simulink model "Basic_3DoF_Delta_2021a"  (R2021a)
settings: Solver=ode4  StartTime=0.0  StopTime=time(end)  FixedStep=0.001  RelTol=1e-6
model workspace: external: MATLAB File robot_6kg_v4_EXa5_DataFile.m (data not in the file)
values from neighbouring files (symbols this model uses):
  IAB = (Im + IA + IB)    [Basic_3DoF_Delta_Dynamic_Param.m]    (also in RL5_6kg_Dynamic_Param.m)
  IABe = (Im + IA + IBe)    [Basic_3DoF_Delta_Dynamic_Param.m]
  lB = l1*(rho1*m1 + me)    [Basic_3DoF_Delta_Dynamic_Param.m]    (also in RL5_6kg_Dynamic_Param.m)
  lBe = l1*(m1/2 + me)    [Basic_3DoF_Delta_Dynamic_Param.m]
  mD = m3 + 3*m2 + 3*me    [Basic_3DoF_Delta_Dynamic_Param.m]    (also in RL5_6kg_Dynamic_Param.m = m3 + 3*m2 + 3*me + mls_a4_spi + mls_a5_spi + mls_a5_worm)
  rho2 = Sro2    [Basic_3DoF_Delta_Dynamic_Param.m]    (also in RL5_6kg_Dynamic_Param.m)
undefined symbols (not defined in the file or in its folder): Inertias, X, Y, Z
libraries: sm_lib x119, nesl_utility x19, eeGeneralControl x3, simulink x3
(part 4 of 4)

== system Basic_3DoF_Delta_2021a/RL5_1450_6kg_Delta_robot_3DoF_Version/a16_pin2 _RIGID ==
  ReferenceFrame : sm_lib/Frames and Transforms/Reference Frame
  Solid(4) : sm_lib/Body Elements/File Solid  Description=Pin  ExtGeomFileName=a16_pin.stp  UnitType=FromFile  ExtGeomFileUnits=m  StepReaderType=HEX  ExportConvexHullGeometry=off  InertiaType=Custom  Mass=Inertias.Solid(4).mass  MassUnits=kg  CenterOfMass=Inertias.Solid(4).CoM  CenterOfMassUnits=m  MomentsOfInertia=Inertias.Solid(4).MoI  MomentsOfInertiaUnits=kg*m^2  ProductsOfInertia=Inertias.Solid(4).PoI  ProductsOfInertiaUnits=kg*m^2  BasedOnType=Density  Density=7850  DensityUnits=kg/m^3  DoExposeReferenceFrame=on  SerializedFrames=<Frames/>  GraphicType=FromGeometry  MarkerShape=Sphere  MarkerSize=10  GraphicVisPropType=SimpleVisualProperties  GraphicDiffuseColor=[0.8 0.8 0.8]  GraphicSpecularColor=[0.5 0.5 0.5 1.0]  GraphicAmbientColor=[0.15 0.15 0.15 1.0]  GraphicEmissiveColor=[0.0 0.0 0.0 1.0]  GraphicShininess=75  GraphicOpacity=1
      settings: AttributesFormatString=|
      | "%<Description>"
      | Mass: %<Mass> [%<MassUnits>]
      | CoM: %<CenterOfMass> [%<CenterOfMassUnits>]
      | MoI: %<MomentsOfInertia> [%<MomentsOfInertiaUnits>]
      | PoI: %<ProductsOfInertia> [%<ProductsOfInertiaUnits>]
  Transform : sm_lib/Frames and Transforms/Rigid Transform  TranslationMethod=StandardAxis  TranslationStandardOffset=67.5  TranslationLengthUnit=mm  TranslationStandardAxis=+X  TranslationCartesianOffset=0  TranslationROffset=0  TranslationROffsetUnits=m  TranslationZOffset=0  TranslationZOffsetUnits=m  TranslationThetaOffset=0  TranslationThetaOffsetUnits=deg  RotationMethod=StandardAxis  RotationAngleUnits=rad  RotationStandardAxis=+Z  RotationAngle=0  RotationArbitraryAxis=0  FollAlignAxisA=+X  BaseAlignAxisA=+Y  FollAlignAxisB=+Y  BaseAlignAxisB=+Z  RotationSequenceAxes=FollowerAxes  RotationSequence=XYX  RotationSequenceAngles=[0 0 0]  RotationSequenceAnglesUnits=deg  RotationMatrix=[1 0 0; 0 1 0; 0 0 1]
  Transform1 : sm_lib/Frames and Transforms/Rigid Transform  TranslationMethod=StandardAxis  TranslationStandardOffset=67.5  TranslationLengthUnit=mm  TranslationStandardAxis=-X  TranslationCartesianOffset=0  TranslationROffset=0  TranslationROffsetUnits=m  TranslationZOffset=0  TranslationZOffsetUnits=m  TranslationThetaOffset=0  TranslationThetaOffsetUnits=deg  RotationMethod=StandardAxis  RotationAngleUnits=deg  RotationStandardAxis=+Y  RotationAngle=180  RotationArbitraryAxis=0  FollAlignAxisA=+X  BaseAlignAxisA=+Y  FollAlignAxisB=+Y  BaseAlignAxisB=+Z  RotationSequenceAxes=FollowerAxes  RotationSequence=XYX  RotationSequenceAngles=[0 0 0]  RotationSequenceAnglesUnits=deg  RotationMatrix=[1 0 0; 0 1 0; 0 0 1]
  Transform2 : sm_lib/Frames and Transforms/Rigid Transform  TranslationMethod=None  TranslationStandardOffset=0  TranslationLengthUnit=mm  TranslationStandardAxis=+Z  TranslationCartesianOffset=0  TranslationROffset=0  TranslationROffsetUnits=m  TranslationZOffset=0  TranslationZOffsetUnits=m  TranslationThetaOffset=0  TranslationThetaOffsetUnits=deg  RotationMethod=StandardAxis  RotationAngleUnits=deg  RotationStandardAxis=+Y  RotationAngle=90  RotationArbitraryAxis=0  FollAlignAxisA=+X  BaseAlignAxisA=+Y  FollAlignAxisB=+Y  BaseAlignAxisB=+Z  RotationSequenceAxes=FollowerAxes  RotationSequence=XYX  RotationSequenceAngles=[0 0 0]  RotationSequenceAnglesUnits=deg  RotationMatrix=[1 0 0; 0 1 0; 0 0 1]
  Center : PMIOPort  Side=Right
  Link 1 : PMIOPort  Port=2  Side=Left
  Link 2 : PMIOPort  Port=3  Side=Left
  connections:
  Transform2/RConn1 -- Center/RConn1
  Transform1/RConn1 -- Link 2/RConn1
  Transform/RConn1 -- Link 1/RConn1
  Transform1/LConn1 -- Solid(4)/RConn1 -- Transform/LConn1 -- ReferenceFrame/RConn1 -- Transform2/LConn1

== system Basic_3DoF_Delta_2021a/RL5_1450_6kg_Delta_robot_3DoF_Version/a16_pin3 _RIGID ==
  ReferenceFrame : sm_lib/Frames and Transforms/Reference Frame
  Solid(4) : sm_lib/Body Elements/File Solid  Description=Pin  ExtGeomFileName=a16_pin.stp  UnitType=FromFile  ExtGeomFileUnits=m  StepReaderType=HEX  ExportConvexHullGeometry=off  InertiaType=Custom  Mass=Inertias.Solid(4).mass  MassUnits=kg  CenterOfMass=Inertias.Solid(4).CoM  CenterOfMassUnits=m  MomentsOfInertia=Inertias.Solid(4).MoI  MomentsOfInertiaUnits=kg*m^2  ProductsOfInertia=Inertias.Solid(4).PoI  ProductsOfInertiaUnits=kg*m^2  BasedOnType=Density  Density=7850  DensityUnits=kg/m^3  DoExposeReferenceFrame=on  SerializedFrames=<Frames/>  GraphicType=FromGeometry  MarkerShape=Sphere  MarkerSize=10  GraphicVisPropType=SimpleVisualProperties  GraphicDiffuseColor=[0.8 0.8 0.8]  GraphicSpecularColor=[0.5 0.5 0.5 1.0]  GraphicAmbientColor=[0.15 0.15 0.15 1.0]  GraphicEmissiveColor=[0.0 0.0 0.0 1.0]  GraphicShininess=75  GraphicOpacity=1
      settings: AttributesFormatString=|
      | "%<Description>"
      | Mass: %<Mass> [%<MassUnits>]
      | CoM: %<CenterOfMass> [%<CenterOfMassUnits>]
      | MoI: %<MomentsOfInertia> [%<MomentsOfInertiaUnits>]
      | PoI: %<ProductsOfInertia> [%<ProductsOfInertiaUnits>]
  Transform : sm_lib/Frames and Transforms/Rigid Transform  TranslationMethod=StandardAxis  TranslationStandardOffset=67.5  TranslationLengthUnit=mm  TranslationStandardAxis=+X  TranslationCartesianOffset=0  TranslationROffset=0  TranslationROffsetUnits=m  TranslationZOffset=0  TranslationZOffsetUnits=m  TranslationThetaOffset=0  TranslationThetaOffsetUnits=deg  RotationMethod=StandardAxis  RotationAngleUnits=rad  RotationStandardAxis=+Z  RotationAngle=0  RotationArbitraryAxis=0  FollAlignAxisA=+X  BaseAlignAxisA=+Y  FollAlignAxisB=+Y  BaseAlignAxisB=+Z  RotationSequenceAxes=FollowerAxes  RotationSequence=XYX  RotationSequenceAngles=[0 0 0]  RotationSequenceAnglesUnits=deg  RotationMatrix=[1 0 0; 0 1 0; 0 0 1]
  Transform1 : sm_lib/Frames and Transforms/Rigid Transform  TranslationMethod=StandardAxis  TranslationStandardOffset=67.5  TranslationLengthUnit=mm  TranslationStandardAxis=-X  TranslationCartesianOffset=0  TranslationROffset=0  TranslationROffsetUnits=m  TranslationZOffset=0  TranslationZOffsetUnits=m  TranslationThetaOffset=0  TranslationThetaOffsetUnits=deg  RotationMethod=StandardAxis  RotationAngleUnits=deg  RotationStandardAxis=+Y  RotationAngle=180  RotationArbitraryAxis=0  FollAlignAxisA=+X  BaseAlignAxisA=+Y  FollAlignAxisB=+Y  BaseAlignAxisB=+Z  RotationSequenceAxes=FollowerAxes  RotationSequence=XYX  RotationSequenceAngles=[0 0 0]  RotationSequenceAnglesUnits=deg  RotationMatrix=[1 0 0; 0 1 0; 0 0 1]
  Transform2 : sm_lib/Frames and Transforms/Rigid Transform  TranslationMethod=None  TranslationStandardOffset=0  TranslationLengthUnit=mm  TranslationStandardAxis=+Z  TranslationCartesianOffset=0  TranslationROffset=0  TranslationROffsetUnits=m  TranslationZOffset=0  TranslationZOffsetUnits=m  TranslationThetaOffset=0  TranslationThetaOffsetUnits=deg  RotationMethod=StandardAxis  RotationAngleUnits=deg  RotationStandardAxis=+Y  RotationAngle=90  RotationArbitraryAxis=0  FollAlignAxisA=+X  BaseAlignAxisA=+Y  FollAlignAxisB=+Y  BaseAlignAxisB=+Z  RotationSequenceAxes=FollowerAxes  RotationSequence=XYX  RotationSequenceAngles=[0 0 0]  RotationSequenceAnglesUnits=deg  RotationMatrix=[1 0 0; 0 1 0; 0 0 1]
  Center : PMIOPort  Side=Left
  Link 1 : PMIOPort  Port=2  Side=Right
  Link 2 : PMIOPort  Port=3  Side=Right
  connections:
  Transform2/RConn1 -- Center/RConn1
  Transform1/RConn1 -- Link 1/RConn1
  Transform/RConn1 -- Link 2/RConn1
  Transform/LConn1 -- Transform1/LConn1 -- Transform2/LConn1 -- Solid(4)/RConn1 -- ReferenceFrame/RConn1

== system Basic_3DoF_Delta_2021a/RL5_1450_6kg_Delta_robot_3DoF_Version/a16_pin4 _RIGID ==
  ReferenceFrame : sm_lib/Frames and Transforms/Reference Frame
  Solid(4) : sm_lib/Body Elements/File Solid  Description=Pin  ExtGeomFileName=a16_pin.stp  UnitType=FromFile  ExtGeomFileUnits=m  StepReaderType=HEX  ExportConvexHullGeometry=off  InertiaType=Custom  Mass=Inertias.Solid(4).mass  MassUnits=kg  CenterOfMass=Inertias.Solid(4).CoM  CenterOfMassUnits=m  MomentsOfInertia=Inertias.Solid(4).MoI  MomentsOfInertiaUnits=kg*m^2  ProductsOfInertia=Inertias.Solid(4).PoI  ProductsOfInertiaUnits=kg*m^2  BasedOnType=Density  Density=7850  DensityUnits=kg/m^3  DoExposeReferenceFrame=on  SerializedFrames=<Frames/>  GraphicType=FromGeometry  MarkerShape=Sphere  MarkerSize=10  GraphicVisPropType=SimpleVisualProperties  GraphicDiffuseColor=[0.8 0.8 0.8]  GraphicSpecularColor=[0.5 0.5 0.5 1.0]  GraphicAmbientColor=[0.15 0.15 0.15 1.0]  GraphicEmissiveColor=[0.0 0.0 0.0 1.0]  GraphicShininess=75  GraphicOpacity=1
      settings: AttributesFormatString=|
      | "%<Description>"
      | Mass: %<Mass> [%<MassUnits>]
      | CoM: %<CenterOfMass> [%<CenterOfMassUnits>]
      | MoI: %<MomentsOfInertia> [%<MomentsOfInertiaUnits>]
      | PoI: %<ProductsOfInertia> [%<ProductsOfInertiaUnits>]
  Transform : sm_lib/Frames and Transforms/Rigid Transform  TranslationMethod=StandardAxis  TranslationStandardOffset=67.5  TranslationLengthUnit=mm  TranslationStandardAxis=+X  TranslationCartesianOffset=0  TranslationROffset=0  TranslationROffsetUnits=m  TranslationZOffset=0  TranslationZOffsetUnits=m  TranslationThetaOffset=0  TranslationThetaOffsetUnits=deg  RotationMethod=StandardAxis  RotationAngleUnits=rad  RotationStandardAxis=+Z  RotationAngle=0  RotationArbitraryAxis=0  FollAlignAxisA=+X  BaseAlignAxisA=+Y  FollAlignAxisB=+Y  BaseAlignAxisB=+Z  RotationSequenceAxes=FollowerAxes  RotationSequence=XYX  RotationSequenceAngles=[0 0 0]  RotationSequenceAnglesUnits=deg  RotationMatrix=[1 0 0; 0 1 0; 0 0 1]
  Transform1 : sm_lib/Frames and Transforms/Rigid Transform  TranslationMethod=StandardAxis  TranslationStandardOffset=67.5  TranslationLengthUnit=mm  TranslationStandardAxis=-X  TranslationCartesianOffset=0  TranslationROffset=0  TranslationROffsetUnits=m  TranslationZOffset=0  TranslationZOffsetUnits=m  TranslationThetaOffset=0  TranslationThetaOffsetUnits=deg  RotationMethod=StandardAxis  RotationAngleUnits=deg  RotationStandardAxis=+Y  RotationAngle=180  RotationArbitraryAxis=0  FollAlignAxisA=+X  BaseAlignAxisA=+Y  FollAlignAxisB=+Y  BaseAlignAxisB=+Z  RotationSequenceAxes=FollowerAxes  RotationSequence=XYX  RotationSequenceAngles=[0 0 0]  RotationSequenceAnglesUnits=deg  RotationMatrix=[1 0 0; 0 1 0; 0 0 1]
  Transform2 : sm_lib/Frames and Transforms/Rigid Transform  TranslationMethod=None  TranslationStandardOffset=0  TranslationLengthUnit=mm  TranslationStandardAxis=+Z  TranslationCartesianOffset=0  TranslationROffset=0  TranslationROffsetUnits=m  TranslationZOffset=0  TranslationZOffsetUnits=m  TranslationThetaOffset=0  TranslationThetaOffsetUnits=deg  RotationMethod=StandardAxis  RotationAngleUnits=deg  RotationStandardAxis=+Y  RotationAngle=90  RotationArbitraryAxis=0  FollAlignAxisA=+X  BaseAlignAxisA=+Y  FollAlignAxisB=+Y  BaseAlignAxisB=+Z  RotationSequenceAxes=FollowerAxes  RotationSequence=XYX  RotationSequenceAngles=[0 0 0]  RotationSequenceAnglesUnits=deg  RotationMatrix=[1 0 0; 0 1 0; 0 0 1]
  Center : PMIOPort  Side=Right
  Link 1 : PMIOPort  Port=2  Side=Left
  Link 2 : PMIOPort  Port=3  Side=Left
  connections:
  Transform2/RConn1 -- Center/RConn1
  Transform1/RConn1 -- Link 2/RConn1
  Transform/RConn1 -- Link 1/RConn1
  Solid(4)/RConn1 -- Transform1/LConn1 -- Transform/LConn1 -- ReferenceFrame/RConn1 -- Transform2/LConn1

== system Basic_3DoF_Delta_2021a/RL5_1450_6kg_Delta_robot_3DoF_Version/a16_pin5 _RIGID ==
  ReferenceFrame : sm_lib/Frames and Transforms/Reference Frame
  Solid(4) : sm_lib/Body Elements/File Solid  Description=Pin  ExtGeomFileName=a16_pin.stp  UnitType=FromFile  ExtGeomFileUnits=m  StepReaderType=HEX  ExportConvexHullGeometry=off  InertiaType=Custom  Mass=Inertias.Solid(4).mass  MassUnits=kg  CenterOfMass=Inertias.Solid(4).CoM  CenterOfMassUnits=m  MomentsOfInertia=Inertias.Solid(4).MoI  MomentsOfInertiaUnits=kg*m^2  ProductsOfInertia=Inertias.Solid(4).PoI  ProductsOfInertiaUnits=kg*m^2  BasedOnType=Density  Density=7850  DensityUnits=kg/m^3  DoExposeReferenceFrame=on  SerializedFrames=<Frames/>  GraphicType=FromGeometry  MarkerShape=Sphere  MarkerSize=10  GraphicVisPropType=SimpleVisualProperties  GraphicDiffuseColor=[0.8 0.8 0.8]  GraphicSpecularColor=[0.5 0.5 0.5 1.0]  GraphicAmbientColor=[0.15 0.15 0.15 1.0]  GraphicEmissiveColor=[0.0 0.0 0.0 1.0]  GraphicShininess=75  GraphicOpacity=1
      settings: AttributesFormatString=|
      | "%<Description>"
      | Mass: %<Mass> [%<MassUnits>]
      | CoM: %<CenterOfMass> [%<CenterOfMassUnits>]
      | MoI: %<MomentsOfInertia> [%<MomentsOfInertiaUnits>]
      | PoI: %<ProductsOfInertia> [%<ProductsOfInertiaUnits>]
  Transform : sm_lib/Frames and Transforms/Rigid Transform  TranslationMethod=StandardAxis  TranslationStandardOffset=67.5  TranslationLengthUnit=mm  TranslationStandardAxis=+X  TranslationCartesianOffset=0  TranslationROffset=0  TranslationROffsetUnits=m  TranslationZOffset=0  TranslationZOffsetUnits=m  TranslationThetaOffset=0  TranslationThetaOffsetUnits=deg  RotationMethod=StandardAxis  RotationAngleUnits=rad  RotationStandardAxis=+Z  RotationAngle=0  RotationArbitraryAxis=0  FollAlignAxisA=+X  BaseAlignAxisA=+Y  FollAlignAxisB=+Y  BaseAlignAxisB=+Z  RotationSequenceAxes=FollowerAxes  RotationSequence=XYX  RotationSequenceAngles=[0 0 0]  RotationSequenceAnglesUnits=deg  RotationMatrix=[1 0 0; 0 1 0; 0 0 1]
  Transform1 : sm_lib/Frames and Transforms/Rigid Transform  TranslationMethod=StandardAxis  TranslationStandardOffset=67.5  TranslationLengthUnit=mm  TranslationStandardAxis=-X  TranslationCartesianOffset=0  TranslationROffset=0  TranslationROffsetUnits=m  TranslationZOffset=0  TranslationZOffsetUnits=m  TranslationThetaOffset=0  TranslationThetaOffsetUnits=deg  RotationMethod=StandardAxis  RotationAngleUnits=deg  RotationStandardAxis=+Y  RotationAngle=180  RotationArbitraryAxis=0  FollAlignAxisA=+X  BaseAlignAxisA=+Y  FollAlignAxisB=+Y  BaseAlignAxisB=+Z  RotationSequenceAxes=FollowerAxes  RotationSequence=XYX  RotationSequenceAngles=[0 0 0]  RotationSequenceAnglesUnits=deg  RotationMatrix=[1 0 0; 0 1 0; 0 0 1]
  Transform2 : sm_lib/Frames and Transforms/Rigid Transform  TranslationMethod=None  TranslationStandardOffset=0  TranslationLengthUnit=mm  TranslationStandardAxis=+Z  TranslationCartesianOffset=0  TranslationROffset=0  TranslationROffsetUnits=m  TranslationZOffset=0  TranslationZOffsetUnits=m  TranslationThetaOffset=0  TranslationThetaOffsetUnits=deg  RotationMethod=StandardAxis  RotationAngleUnits=deg  RotationStandardAxis=+Y  RotationAngle=90  RotationArbitraryAxis=0  FollAlignAxisA=+X  BaseAlignAxisA=+Y  FollAlignAxisB=+Y  BaseAlignAxisB=+Z  RotationSequenceAxes=FollowerAxes  RotationSequence=XYX  RotationSequenceAngles=[0 0 0]  RotationSequenceAnglesUnits=deg  RotationMatrix=[1 0 0; 0 1 0; 0 0 1]
  Center : PMIOPort  Side=Left
  Link 1 : PMIOPort  Port=2  Side=Right
  Link 2 : PMIOPort  Port=3  Side=Right
  connections:
  Transform2/RConn1 -- Center/RConn1
  Transform1/RConn1 -- Link 1/RConn1
  Transform/RConn1 -- Link 2/RConn1
  Transform/LConn1 -- Transform1/LConn1 -- Transform2/LConn1 -- Solid(4)/RConn1 -- ReferenceFrame/RConn1

== system Basic_3DoF_Delta_2021a/RL5_1450_6kg_Delta_robot_3DoF_Version/a16_pin6 _RIGID ==
  ReferenceFrame : sm_lib/Frames and Transforms/Reference Frame
  Solid(4) : sm_lib/Body Elements/File Solid  Description=Pin  ExtGeomFileName=a16_pin.stp  UnitType=FromFile  ExtGeomFileUnits=m  StepReaderType=HEX  ExportConvexHullGeometry=off  InertiaType=Custom  Mass=Inertias.Solid(4).mass  MassUnits=kg  CenterOfMass=Inertias.Solid(4).CoM  CenterOfMassUnits=m  MomentsOfInertia=Inertias.Solid(4).MoI  MomentsOfInertiaUnits=kg*m^2  ProductsOfInertia=Inertias.Solid(4).PoI  ProductsOfInertiaUnits=kg*m^2  BasedOnType=Density  Density=7850  DensityUnits=kg/m^3  DoExposeReferenceFrame=on  SerializedFrames=<Frames/>  GraphicType=FromGeometry  MarkerShape=Sphere  MarkerSize=10  GraphicVisPropType=SimpleVisualProperties  GraphicDiffuseColor=[0.8 0.8 0.8]  GraphicSpecularColor=[0.5 0.5 0.5 1.0]  GraphicAmbientColor=[0.15 0.15 0.15 1.0]  GraphicEmissiveColor=[0.0 0.0 0.0 1.0]  GraphicShininess=75  GraphicOpacity=1
      settings: AttributesFormatString=|
      | "%<Description>"
      | Mass: %<Mass> [%<MassUnits>]
      | CoM: %<CenterOfMass> [%<CenterOfMassUnits>]
      | MoI: %<MomentsOfInertia> [%<MomentsOfInertiaUnits>]
      | PoI: %<ProductsOfInertia> [%<ProductsOfInertiaUnits>]
  Transform : sm_lib/Frames and Transforms/Rigid Transform  TranslationMethod=StandardAxis  TranslationStandardOffset=67.5  TranslationLengthUnit=mm  TranslationStandardAxis=+X  TranslationCartesianOffset=0  TranslationROffset=0  TranslationROffsetUnits=m  TranslationZOffset=0  TranslationZOffsetUnits=m  TranslationThetaOffset=0  TranslationThetaOffsetUnits=deg  RotationMethod=StandardAxis  RotationAngleUnits=rad  RotationStandardAxis=+Z  RotationAngle=0  RotationArbitraryAxis=0  FollAlignAxisA=+X  BaseAlignAxisA=+Y  FollAlignAxisB=+Y  BaseAlignAxisB=+Z  RotationSequenceAxes=FollowerAxes  RotationSequence=XYX  RotationSequenceAngles=[0 0 0]  RotationSequenceAnglesUnits=deg  RotationMatrix=[1 0 0; 0 1 0; 0 0 1]
  Transform1 : sm_lib/Frames and Transforms/Rigid Transform  TranslationMethod=StandardAxis  TranslationStandardOffset=67.5  TranslationLengthUnit=mm  TranslationStandardAxis=-X  TranslationCartesianOffset=0  TranslationROffset=0  TranslationROffsetUnits=m  TranslationZOffset=0  TranslationZOffsetUnits=m  TranslationThetaOffset=0  TranslationThetaOffsetUnits=deg  RotationMethod=StandardAxis  RotationAngleUnits=deg  RotationStandardAxis=+Y  RotationAngle=180  RotationArbitraryAxis=0  FollAlignAxisA=+X  BaseAlignAxisA=+Y  FollAlignAxisB=+Y  BaseAlignAxisB=+Z  RotationSequenceAxes=FollowerAxes  RotationSequence=XYX  RotationSequenceAngles=[0 0 0]  RotationSequenceAnglesUnits=deg  RotationMatrix=[1 0 0; 0 1 0; 0 0 1]
  Transform2 : sm_lib/Frames and Transforms/Rigid Transform  TranslationMethod=None  TranslationStandardOffset=0  TranslationLengthUnit=mm  TranslationStandardAxis=+Z  TranslationCartesianOffset=0  TranslationROffset=0  TranslationROffsetUnits=m  TranslationZOffset=0  TranslationZOffsetUnits=m  TranslationThetaOffset=0  TranslationThetaOffsetUnits=deg  RotationMethod=StandardAxis  RotationAngleUnits=deg  RotationStandardAxis=+Y  RotationAngle=90  RotationArbitraryAxis=0  FollAlignAxisA=+X  BaseAlignAxisA=+Y  FollAlignAxisB=+Y  BaseAlignAxisB=+Z  RotationSequenceAxes=FollowerAxes  RotationSequence=XYX  RotationSequenceAngles=[0 0 0]  RotationSequenceAnglesUnits=deg  RotationMatrix=[1 0 0; 0 1 0; 0 0 1]
  Center : PMIOPort  Side=Right
  Link 1 : PMIOPort  Port=2  Side=Left
  Link 2 : PMIOPort  Port=3  Side=Left
  connections:
  Transform2/RConn1 -- Center/RConn1
  Transform1/RConn1 -- Link 2/RConn1
  Transform/RConn1 -- Link 1/RConn1
  Solid(4)/RConn1 -- Transform1/LConn1 -- Transform/LConn1 -- ReferenceFrame/RConn1 -- Transform2/LConn1

== matlab function Basic_3DoF_Delta_2021a/Dynamic Model ==
  data: Psi output; dD input; D input; q input; dq input; ddq input; dynpar input; tau_cp output; tau_ce output
function [Psi,tau_cp,tau_ce] = dyn(dD,D,q,dq,ddq,dynpar)
% This function block represents mathematical DYNAMIC MODEL for Basic 3-DoF Delta 

q0 = 5.327998*pi/180;   % [rad], 5.327998° ~ q0*pi/180 rad, angle( axis_i & line(A_i,B_i) )
r0 =  0.330;            % [m], radius of circumscribed circle of equilat. basic frame triangle
l1 =  0.420;            % [m], lengths of upper arms
% l2 =  1.055;          % [m], lengths of forearms, not used
r3 =  0.125;            % [m], radius of circumscribed circle of equilat. mov. platform trngl.
% r4 =  0.0632;         % [m], radius of wrist arm offset, distance from point E to F
% r4m = 0.0424798;      % [m], radius of wrist arm CoG point offset,distance from point E to \bar{F} 
% h4 =  0.132;          % [m], perpendicular distance from point D to E (h4m = h4), not used
% r5 =  0.135;          % [m], radius of swivel arm (distance A5-axis vs. Tool Center Point (TCP)), not used
% r5m = 0.1225 - 0.0432725;     % distance from F to the CoG of the swivel arm; translation in Z = 0.1225, Inertias.Solid(11).CoM(3)=0.0432725. 
dr =  r0 - r3;                  % [m], useful simplifying constant

% Actuated joint positions
q1 = q(1) - q0; q2 = q(2) - q0;  q3 = q(3) - q0;    % q4 = q(4);  q5 = q(5);

% Actuated joint velocities
dq1 = dq(1);  dq2 = dq(2);  dq3 = dq(3);            % dq4 = dq(4);  dq5 = dq(5);

% Actuated joint accelerations
ddq1 = ddq(1);  ddq2 = ddq(2);  ddq3 = ddq(3);      % ddq4 = ddq(4);  ddq5 = ddq(5);

% Point D positions
xD = D(1);  yD = D(2);  zD = D(3); 

% Point D velocities
dxD = dD(1);  dyD = dD(2);  dzD = dD(3);

%% Dynamic model mass parameters
g = 9.80665;        % [m]/s^2, gravity

mD = dynpar(1);     % Constant total mass at movable platform level (point D)

%% Jacobian matrices J_D, J_q, J_\mathcal{D} and their derivatives and inverses

[Jd,Jq] = Jcq(xD,yD,zD,dr,l1,q1,q2,q3);             % Eq (20) in the paper: Jd = J_D, Jq = J_q 
Jqd = Jd\Jq; iJqd = Jq\Jd;                          % Eq (21) in the paper: Jqd = J_qD, iJqd = J_qD^{-1}

JD = [Jqd, zeros(3,2); zeros(2,3), eye(2)];         % Eq (22) in the paper: JD = J_\mathcal{D}

[dJc,dJq] = dJcq(xD,yD,zD,dxD,dyD,dzD,dr,l1,q1,q2,q3,dq1,dq2,dq3); 
dJqd = Jd\(dJq-dJc*Jqd);                            % Eq (25) in the paper: derivative of J_qD

dJD = [dJqd, zeros(3,2) ; zeros(2,3), zeros(2)];    % derivative of J_\mathcal{D}

%% Dynamical model of the parallel part (A1-A2-A3): Equation of Motion: Eq. (40) with (51)

ld = sqrt(xD^2+yD^2);                   % distance of point D inn XY plane from point O

m2 = 1.05;
rho2 = dynpar(2);                       % mass distribution ratio for upper arms 
rho2e = 2/3;                            % in Codourey'96

mD =  mD - ( rho2*m2*(cos(q1)+cos(q2)+cos(q3)) );    % the mass of the movable platform with trajectoryy-dependent contribution of forearm masses
mDe = mD - 2*m2;                                     % in Codourey'96

IAB = dynpar(3);                                     % fixed inertia values of each upper arm excluding the effect of m2
IAB = diag([IAB + l1^2*rho2*cos(q1)*m2, IAB + l1^2*rho2*cos(q2)*m2, IAB + l1^2*rho2*cos(q3)*m2, 0, 0]); % inertia matrix for upper arms 
IABe = dynpar(5);                                    % in Codourey'96
IABe = diag([IABe + l1^2*rho2e*m2, IABe + l1^2*rho2e*m2, IABe + l1^2*rho2e*m2, 0, 0]); % in Codourey'96

I_35 = [eye(3), zeros(3,2)];
Ma = I_35*( IAB + mD*(JD'*JD) );        % Eq. (51) in the paper: Inertial matrix for the parallel part
Mae = I_35*( IABe + mDe*(JD'*JD) );     % in Codourey'96

Ca = I_35*( mD*JD'*dJD ) ;              % Eq. (51) in the paper: Coriolis & centrifugal matrix for the parallel part
Cae = I_35*( mDe*JD'*dJD ) ;            % in Codourey'96

lBnum = dynpar(4);
lBnume = dynpar(6); 

Ga = I_35*diag([lBnum + l1*rho2*cos(q1)*m2, lBnum + l1*rho2*cos(q2)*m2, lBnum + l1*rho2*cos(q3)*m2, 0, 0])*g*[cos(q1); cos(q2); cos(q3); 0; 0] ...
   - I_35*( mD*JD' )*[0; 0; -g; 0; 0] ;      % Eq. (51) with (48) in the paper: Gravitational matrix for the parallel part
Gae = I_35*diag([lBnume + l1*rho2e*m2, lBnume + l1*rho2e*m2, lBnume + l1*rho2e*m2, 0, 0])*g*[cos(q1); cos(q2); cos(q3); 0; 0] ...
   - I_35*( mDe*JD' )*[0; 0; -g; 0; 0] ;     % in Codourey'96


tau_ap = Ma*ddq + Ca*dq + Ga ;                                   % Torque vector of the actuated upper arms with proposed model
tau_ae = Mae*ddq + Cae*dq + Gae ;                                % with Coudrey'96 model

%% Collecting data for the regressor matrix (64) of the regression model from the sampled values of (62)
Sig10 = ddq1; 
% Sig14 = g*JF(3,1) + dq1*(dJF(1,1)*JF(1,1) + dJF(2,1)*JF(2,1) + dJF(3,1)*JF(3,1) + dJF(4,1)*JF(4,1)) + dq2*(dJF(1,2)*JF(1,1) + dJF(2,2)*JF(2,1) + dJF(3,2)*JF(3,1) + dJF(4,2)*JF(4,1)) + dq3*(dJF(1,3)*JF(1,1) + dJF(2,3)*JF(2,1) + dJF(3,3)*JF(3,1) + dJF(4,3)*JF(4,1)) + dq4*(dJF(1,4)*JF(1,1) + dJF(2,4)*JF(2,1) + dJF(3,4)*JF(3,1) + dJF(4,4)*JF(4,1)) + ddq1*(JF (1,1)^2 + JF (2,1)^2 + JF (3,1)^2 + JF (4,1)^2) + ddq2*(JF(1,1)*JF(1,2) + JF(2,1)*JF(2,2) + JF(3,1)*JF(3,2) + JF(4,1)*JF(4,2)) + ddq3*(JF(1,1)*JF(1,3) + JF(2,1)*JF(2,3) + JF(3,1)*JF(3,3) + JF(4,1)*JF(4,3)) + ddq4*(JF(1,1)*JF(1,4) + JF(2,1)*JF(2,4) + JF(3,1)*JF(3,4) + JF(4,1)*JF(4,4));
Sig14 = 0;      % due excluding wrist arm, i.e. m4=0
% Sig15 = g*JH(3,1) + dq1*(dJH(1,1)*JH(1,1) + dJH(2,1)*JH(2,1) + dJH(3,1)*JH(3,1) + dJH(4,1)*JH(4,1) + dJH(5,1)*JH(5,1)) + dq2*(dJH(1,2)*JH(1,1) + dJH(2,2)*JH(2,1) + dJH(3,2)*JH(3,1) + dJH(4,2)*JH(4,1) + dJH(5,2)*JH(5,1)) + dq3*(dJH(1,3)*JH(1,1) + dJH(2,3)*JH(2,1) + dJH(3,3)*JH(3,1) + dJH(4,3)*JH(4,1) + dJH(5,3)*JH(5,1)) + dq4*(dJH(1,4)*JH(1,1) + dJH(2,4)*JH(2,1) + dJH(3,4)*JH(3,1) + dJH(4,4)*JH(4,1) + dJH(5,4)*JH(5,1)) + dq5*(dJH(1,5)*JH(1,1) + dJH(2,5)*JH(2,1) + dJH(3,5)*JH(3,1) + dJH(4,5)*JH(4,1) + dJH(5,5)*JH(5,1)) + ddq1*(JH (1,1)^2 + JH (2,1)^2 + JH (3,1)^2 + JH (4,1)^2 + JH (5,1)^2) + ddq2*(JH(1,1)*JH(1,2) + JH(2,1)*JH(2,2) + JH(3,1)*JH(3,2) + JH(4,1)*JH(4,2) + JH(5,1)*JH(5,2)) + ddq3*(JH(1,1)*JH(1,3) + JH(2,1)*JH(2,3) + JH(3,1)*JH(3,3) + JH(4,1)*JH(4,3) + JH(5,1)*JH(5,3)) + ddq4*(JH(1,1)*JH(1,4) + JH(2,1)*JH(2,4) + JH(3,1)*JH(3,4) + JH(4,1)*JH(4,4) + JH(5,1)*JH(5,4)) + ddq5*(JH(1,1)*JH(1,5) + JH(2,1)*JH(2,5) + JH(3,1)*JH(3,5) + JH(4,1)*JH(4,5) + JH(5,1)*JH(5,5));
Sig15 = 0;      % due excluding swivel arm, i.e. m5=0
Sig1D = g*JD(3,1) + dq1*(dJqd(1,1)*JD(1,1) + dJqd(2,1)*JD(2,1) + dJqd(3,1)*JD(3,1)) + dq2*(dJqd(1,2)*JD(1,1) + dJqd(2,2)*JD(2,1) + dJqd(3,2)*JD(3,1)) + dq3*(dJqd(1,3)*JD(1,1) + dJqd(2,3)*JD(2,1) + dJqd(3,3)*JD(3,1)) + ddq1*(JD (1,1)^2 + JD (2,1)^2 + JD (3,1)^2) + ddq2*(JD(1,1)*JD(1,2) + JD(2,1)*JD(2,2) + JD(3,1)*JD(3,2)) + ddq3*(JD(1,1)*JD(1,3) + JD(2,1)*JD(2,3) + JD(3,1)*JD(3,3));
% Sig1Ds = g*JD(3,1);
Sig1Ds = 0;     % due excluding shafts, i.e. m6l=m6u=0 or mDs=0
%
Sig20 = ddq2; 
% Sig24 = g*JF(3,2) + dq1*(dJF(1,1)*JF(1,2) + dJF(2,1)*JF(2,2) + dJF(3,1)*JF(3,2) + dJF(4,1)*JF(4,2)) + dq2*(dJF(1,2)*JF(1,2) + dJF(2,2)*JF(2,2) + dJF(3,2)*JF(3,2) + dJF(4,2)*JF(4,2)) + dq3*(dJF(1,3)*JF(1,2) + dJF(2,3)*JF(2,2) + dJF(3,3)*JF(3,2) + dJF(4,3)*JF(4,2)) + dq4*(dJF(1,4)*JF(1,2) + dJF(2,4)*JF(2,2) + dJF(3,4)*JF(3,2) + dJF(4,4)*JF(4,2)) + ddq1*(JF(1,1)*JF(1,2) + JF(2,1)*JF(2,2) + JF(3,1)*JF(3,2) + JF(4,1)*JF(4,2)) + ddq2*(JF (1,2)^2 + JF (2,2)^2 + JF (3,2)^2 + JF (4,2)^2) + ddq3*(JF(1,2)*JF(1,3) + JF(2,2)*JF(2,3) + JF(3,2)*JF(3,3) + JF(4,2)*JF(4,3)) + ddq4*(JF(1,2)*JF(1,4) + JF(2,2)*JF(2,4) + JF(3,2)*JF(3,4) + JF(4,2)*JF(4,4)); 
Sig24 = 0;      % due excluding wrist arm, i.e. m4=0
% Sig25 = g*JH(3,2) + dq1*(dJH(1,1)*JH(1,2) + dJH(2,1)*JH(2,2) + dJH(3,1)*JH(3,2) + dJH(4,1)*JH(4,2) + dJH(5,1)*JH(5,2)) + dq2*(dJH(1,2)*JH(1,2) + dJH(2,2)*JH(2,2) + dJH(3,2)*JH(3,2) + dJH(4,2)*JH(4,2) + dJH(5,2)*JH(5,2)) + dq3*(dJH(1,3)*JH(1,2) + dJH(2,3)*JH(2,2) + dJH(3,3)*JH(3,2) + dJH(4,3)*JH(4,2) + dJH(5,3)*JH(5,2)) + dq4*(dJH(1,4)*JH(1,2) + dJH(2,4)*JH(2,2) + dJH(3,4)*JH(3,2) + dJH(4,4)*JH(4,2) + dJH(5,4)*JH(5,2)) + dq5*(dJH(1,5)*JH(1,2) + dJH(2,5)*JH(2,2) + dJH(3,5)*JH(3,2) + dJH(4,5)*JH(4,2) + dJH(5,5)*JH(5,2)) + ddq1*(JH(1,1)*JH(1,2) + JH(2,1)*JH(2,2) + JH(3,1)*JH(3,2) + JH(4,1)*JH(4,2) + JH(5,1)*JH(5,2)) + ddq2*(JH (1,2)^2 + JH (2,2)^2 + JH (3,2)^2 + JH (4,2)^2 + JH (5,2)^2) + ddq3*(JH(1,2)*JH(1,3) + JH(2,2)*JH(2,3) + JH(3,2)*JH(3,3) + JH(4,2)*JH(4,3) + JH(5,2)*JH(5,3)) + ddq4*(JH(1,2)*JH(1,4) + JH(2,2)*JH(2,4) + JH(3,2)*JH(3,4) + JH(4,2)*JH(4,4) + JH(5,2)*JH(5,4)) + ddq5*(JH(1,2)*JH(1,5) + JH(2,2)*JH(2,5) + JH(3,2)*JH(3,5) + JH(4,2)*JH(4,5) + JH(5,2)*JH(5,5)); 
Sig25 = 0;      % due excluding swivel arm, i.e. m5=0
Sig2D = g*JD(3,2) + dq1*(dJqd(1,1)*JD(1,2) + dJqd(2,1)*JD(2,2) + dJqd(3,1)*JD(3,2)) + dq2*(dJqd(1,2)*JD(1,2) + dJqd(2,2)*JD(2,2) + dJqd(3,2)*JD(3,2)) + dq3*(dJqd(1,3)*JD(1,2) + dJqd(2,3)*JD(2,2) + dJqd(3,3)*JD(3,2)) + ddq1*(JD(1,1)*JD(1,2) + JD(2,1)*JD(2,2) + JD(3,1)*JD(3,2)) + ddq2*(JD (1,2)^2 + JD (2,2)^2 + JD (3,2)^2) + ddq3*(JD(1,2)*JD(1,3) + JD(2,2)*JD(2,3) + JD(3,2)*JD(3,3)); 
% Sig2Ds = g*JD(3,2);
Sig2Ds = 0;     % due excluding shafts, i.e. m6l=m6u=0 or mDs=0
%
Sig30 = ddq3; 
% Sig34 = g*JF(3,3) + dq1*(dJF(1,1)*JF(1,3) + dJF(2,1)*JF(2,3) + dJF(3,1)*JF(3,3) + dJF(4,1)*JF(4,3)) + dq2*(dJF(1,2)*JF(1,3) + dJF(2,2)*JF(2,3) + dJF(3,2)*JF(3,3) + dJF(4,2)*JF(4,3)) + dq3*(dJF(1,3)*JF(1,3) + dJF(2,3)*JF(2,3) + dJF(3,3)*JF(3,3) + dJF(4,3)*JF(4,3)) + dq4*(dJF(1,4)*JF(1,3) + dJF(2,4)*JF(2,3) + dJF(3,4)*JF(3,3) + dJF(4,4)*JF(4,3)) + ddq1*(JF(1,1)*JF(1,3) + JF(2,1)*JF(2,3) + JF(3,1)*JF(3,3) + JF(4,1)*JF(4,3)) + ddq2*(JF(1,2)*JF(1,3) + JF(2,2)*JF(2,3) + JF(3,2)*JF(3,3) + JF(4,2)*JF(4,3)) + ddq3*(JF (1,3)^2 + JF (2,3)^2 + JF (3,3)^2 + JF (4,3)^2) + ddq4*(JF(1,3)*JF(1,4) + JF(2,3)*JF(2,4) + JF(3,3)*JF(3,4) + JF(4,3)*JF(4,4));
Sig34 = 0 ;      % due excluding wrist arm, i.e. m4=0
% Sig35 = g*JH(3,3) + dq1*(dJH(1,1)*JH(1,3) + dJH(2,1)*JH(2,3) + dJH(3,1)*JH(3,3) + dJH(4,1)*JH(4,3) + dJH(5,1)*JH(5,3)) + dq2*(dJH(1,2)*JH(1,3) + dJH(2,2)*JH(2,3) + dJH(3,2)*JH(3,3) + dJH(4,2)*JH(4,3) + dJH(5,2)*JH(5,3)) + dq3*(dJH(1,3)*JH(1,3) + dJH(2,3)*JH(2,3) + dJH(3,3)*JH(3,3) + dJH(4,3)*JH(4,3) + dJH(5,3)*JH(5,3)) + dq4*(dJH(1,4)*JH(1,3) + dJH(2,4)*JH(2,3) + dJH(3,4)*JH(3,3) + dJH(4,4)*JH(4,3) + dJH(5,4)*JH(5,3)) + dq5*(dJH(1,5)*JH(1,3) + dJH(2,5)*JH(2,3) + dJH(3,5)*JH(3,3) + dJH(4,5)*JH(4,3) + dJH(5,5)*JH(5,3)) + ddq1*(JH(1,1)*JH(1,3) + JH(2,1)*JH(2,3) + JH(3,1)*JH(3,3) + JH(4,1)*JH(4,3) + JH(5,1)*JH(5,3)) + ddq2*(JH(1,2)*JH(1,3) + JH(2,2)*JH(2,3) + JH(3,2)*JH(3,3) + JH(4,2)*JH(4,3) + JH(5,2)*JH(5,3)) + ddq3*(JH (1,3)^2 + JH (2,3)^2 + JH (3,3)^2 + JH (4,3)^2 + JH (5,3)^2) + ddq4*(JH(1,3)*JH(1,4) + JH(2,3)*JH(2,4) + JH(3,3)*JH(3,4) + JH(4,3)*JH(4,4) + JH(5,3)*JH(5,4)) + ddq5*(JH(1,3)*JH(1,5) + JH(2,3)*JH(2,5) + JH(3,3)*JH(3,5) + JH(4,3)*JH(4,5) + JH(5,3)*JH(5,5));
Sig35 = 0;      % due excluding swivel arm, i.e. m5=0 
Sig3D = g*JD(3,3)+dq1*(dJqd(1,1)*JD(1,3)+dJqd(2,1)*JD(2,3)+dJqd(3,1)*JD(3,3))+dq2*(dJqd(1,2)*JD(1,3)+dJqd(2,2)*JD(2,3)+dJqd(3,2)*JD(3,3))+dq3*(dJqd(1,3)*JD(1,3)+dJqd(2,3)*JD(2,3)+dJqd(3,3)*JD(3,3))+ddq1*(JD(1,1)*JD(1,3)+JD(2,1)*JD(2,3)+JD(3,1)*JD(3,3))+ddq2*(JD(1,2)*JD(1,3)+JD(2,2)*JD(2,3)+JD(3,2)*JD(3,3))+ddq3*(JD (1,3)^2+JD (2,3)^2+JD (3,3)^2); 
% Sig3Ds = g*JD(3,3);
Sig3Ds = 0;     % due excluding shafts, i.e. m6l=m6u=0 or mDs=0
%
Psi = [ Sig10, Sig10*cos(q1), Sig14, Sig15, Sig1D, -Sig1D*(cos(q1)+cos(q2)+cos(q3)), Sig1Ds*ld, Sig1Ds, -Sig1Ds*ld, g*cos(q1), g*(cos(q1))^2 ; ...
        Sig20, Sig20*cos(q2), Sig24, Sig25, Sig2D, -Sig2D*(cos(q1)+cos(q2)+cos(q3)), Sig2Ds*ld, Sig2Ds, -Sig2Ds*ld, g*cos(q2), g*(cos(q2))^2 ; ...
        Sig30, Sig30*cos(q3), Sig34, Sig35, Sig3D, -Sig3D*(cos(q1)+cos(q2)+cos(q3)), Sig3Ds*ld, Sig3Ds, -Sig3Ds*ld, g*cos(q3), g*(cos(q3))^2 ] ;

%% UPPER ARM ACTUATED JOINT TORQUE VECTORS

tau_cp = [tau_ap];      % Eq. (40) in the paper
tau_ce = [tau_ae];      % with Codourey'96 model

end

function [Jc,Jq] = Jcq(xD,yD,zD,dr,l1,q1,q2,q3)
Jc = [ 2*xD - 2*dr - 2*l1*cos(q1), 2*yD, 2*zD - 2*l1*sin(q1); ...
       dr + 2*xD + l1*cos(q2), 2*yD - 3^(1/2)*dr - 3^(1/2)*l1*cos(q2), 2*zD - 2*l1*sin(q2); ...
       dr + 2*xD + l1*cos(q3), 2*yD + 3^(1/2)*dr + 3^(1/2)*l1*cos(q3), 2*zD - 2*l1*sin(q3)];
Jq = [ 2*l1*(dr*sin(q1) + zD*cos(q1) - xD*sin(q1)), 0, 0 ; ...
       0, l1*(2*dr*sin(q2) + 2*zD*cos(q2) + xD*sin(q2) - 3^(1/2)*yD*sin(q2)), 0; ...
       0, 0, l1*(2*dr*sin(q3) + 2*zD*cos(q3) + xD*sin(q3) + 3^(1/2)*yD*sin(q3))];
end

function [dJc,dJq] = dJcq(xD,yD,zD,dxD,dyD,dzD,dr,l1,q1,q2,q3,dq1,dq2,dq3)
dJc = [2*dxD + 2*l1*sin(q1)*dq1, 2*dyD, 2*dzD - 2*l1*cos(q1)*dq1 ; ...
       2*dxD - l1*sin(q2)*dq2, 2*dyD + 3^(1/2)*l1*sin(q2)*dq2, 2*dzD - 2*l1*cos(q2)*dq2 ; ...
       2*dxD - l1*sin(q3)*dq3, 2*dyD - 3^(1/2)*l1*sin(q3)*dq3, 2*dzD - 2*l1*cos(q3)*dq3];
dJq = [-2*l1*(sin(q1)*dxD - cos(q1)*dzD + cos(q1)*xD*dq1 + sin(q1)*zD*dq1 - dr*cos(q1)*dq1), 0, 0 ; ...
        0, l1*(2*cos(q2)*dzD + sin(q2)*dxD + cos(q2)*xD*dq2 - 2*sin(q2)*zD*dq2 + 2*dr*cos(q2)*dq2 - 3^(1/2)*sin(q2)*dyD - 3^(1/2)*cos(q2)*yD*dq2), 0 ; ...
        0, 0, l1*(2*cos(q3)*dzD + sin(q3)*dxD + cos(q3)*xD*dq3 - 2*sin(q3)*zD*dq3 + 2*dr*cos(q3)*dq3 + 3^(1/2)*sin(q3)*dyD + 3^(1/2)*cos(q3)*yD*dq3)];
end

== matlab function Basic_3DoF_Delta_2021a/Kinematic model ==
  data: dD input; D input; q input; dq input; dD_c output; ddq input; ddD_c output
function [dD_c, ddD_c] = kin(dD,D,q,dq,ddq)
% This function block represents FORWARD KINEMATICS FOR VELOCITY 

q0 = 5.327998*pi/180;   % [rad], 5.327998° ~ q0*pi/180 rad, angle( axis_i & line(A_i,B_i) )
r0 =  0.330;            % [m], radius of circumscribed circle of equilat. basic frame triangle
l1 =  0.420;            % [m], lengths of upper arms
% l2 =  1.055;          % [m], lengths of forearms, not used
r3 =  0.125;            % [m], radius of circumscribed circle of equilat. mov. platform trngl.
% r4 =  0.0632;           % [m], radius of wrist arm offset, distance from point E to F
% h4 =  0.132;          % [m], perpendicular distance from point D to E (h4m = h4), not used
% r5 =  0.135;            % [m], radius of swivel arm (distance A5-axis vs. Tool Center Point (TCP)), not used
dr =  r0 - r3;          % [m], useful simplifying constant

% Actuated joint positions
q1 = q(1) - q0; q2 = q(2) - q0;  q3 = q(3) - q0;    % q4 = q(4);  q5 = q(5);

% Actuated joint velocities
dq1 = dq(1);  dq2 = dq(2);  dq3 = dq(3);            % dq4 = dq(4);  dq5 = dq(5);

% Actuated joint accelerations
ddq1 = ddq(1);  ddq2 = ddq(2);  ddq3 = ddq(3);      % ddq4 = ddq(4);  ddq5 = ddq(5);

% Point D position
xD = D(1);  yD = D(2);  zD = D(3); 

% Point D velocity
dxD = dD(1);  dyD = dD(2);  dzD = dD(3);

%% Jacobian matrices J_D, J_q, J_\mathcal{D}, J and their derivatives and inverses

[Jd,Jq] = Jcq(xD,yD,zD,dr,l1,q1,q2,q3);             % Eq (20) in the paper: Jd = J_D, Jq = J_q 
Jqd = Jd\Jq; iJqd = Jq\Jd;                          % Eq (21) in the paper: Jqd = J_qD, iJqd = J_qD^{-1}

[dJc,dJq] = dJcq(xD,yD,zD,dxD,dyD,dzD,dr,l1,q1,q2,q3,dq1,dq2,dq3); 
dJqd = Jd\(dJq-dJc*Jqd);                            % Eq (25) in the paper: derivative of J_qD

%% Calculated point D velocity and acceleration
dD_c = Jqd*[dq1; dq2 ;dq3];                                % Eq. (21) in the paper
ddD_c = dJqd*[dq1; dq2 ;dq3] + Jqd*[ddq1; ddq2 ;ddq3] ;    % Eq. (24) in the paper

end

function [Jc,Jq] = Jcq(xD,yD,zD,dr,l1,q1,q2,q3)
Jc = [ 2*xD - 2*dr - 2*l1*cos(q1),                                   2*yD, 2*zD - 2*l1*sin(q1); ...
       dr + 2*xD + l1*cos(q2), 2*yD - 3^(1/2)*dr - 3^(1/2)*l1*cos(q2), 2*zD - 2*l1*sin(q2); ...
       dr + 2*xD + l1*cos(q3), 2*yD + 3^(1/2)*dr + 3^(1/2)*l1*cos(q3), 2*zD - 2*l1*sin(q3)];
Jq = [ 2*l1*(dr*sin(q1) + zD*cos(q1) - xD*sin(q1)), 0, 0 ; ...
       0, l1*(2*dr*sin(q2) + 2*zD*cos(q2) + xD*sin(q2) - 3^(1/2)*yD*sin(q2)), 0; ...
       0, 0, l1*(2*dr*sin(q3) + 2*zD*cos(q3) + xD*sin(q3) + 3^(1/2)*yD*sin(q3))];
end

function [dJc,dJq] = dJcq(xD,yD,zD,dxD,dyD,dzD,dr,l1,q1,q2,q3,dq1,dq2,dq3)
dJc = [2*dxD + 2*l1*sin(q1)*dq1, 2*dyD, 2*dzD - 2*l1*cos(q1)*dq1 ; ...
       2*dxD - l1*sin(q2)*dq2, 2*dyD + 3^(1/2)*l1*sin(q2)*dq2, 2*dzD - 2*l1*cos(q2)*dq2 ; ...
       2*dxD - l1*sin(q3)*dq3, 2*dyD - 3^(1/2)*l1*sin(q3)*dq3, 2*dzD - 2*l1*cos(q3)*dq3];
dJq = [-2*l1*(sin(q1)*dxD - cos(q1)*dzD + cos(q1)*xD*dq1 + sin(q1)*zD*dq1 - dr*cos(q1)*dq1), 0, 0 ; ...
        0, l1*(2*cos(q2)*dzD + sin(q2)*dxD + cos(q2)*xD*dq2 - 2*sin(q2)*zD*dq2 + 2*dr*cos(q2)*dq2 - 3^(1/2)*sin(q2)*dyD - 3^(1/2)*cos(q2)*yD*dq2), 0 ; ...
        0, 0, l1*(2*cos(q3)*dzD + sin(q3)*dxD + cos(q3)*xD*dq3 - 2*sin(q3)*zD*dq3 + 2*dr*cos(q3)*dq3 + 3^(1/2)*sin(q3)*dyD + 3^(1/2)*cos(q3)*yD*dq3)];
end
